simulink model "BBB_USRLED_v2"  (R2013a)
settings: Solver=FixedStepDiscrete  SolverMode=SingleTasking  StartTime=0.0  StopTime=10.0  RelTol=1e-3
libraries: simulink x1
settings Model: ExtModeTrigDuration=100  Creator=rdustinkahawita  LastModifiedBy=rdustinkahawita
settings DataIOCC: InspectSignalLogs=on
settings OptimizationCC: OptimizeModelRefInitCode=on  LifeSpan=1
settings DebuggingCC: SolverPrmCheckMsg=none  StrictBusMsg=Warning
settings HardwareCC: ProdLargestAtomicInteger=Long  ProdLargestAtomicFloat=Double  ProdEndianess=LittleEndian  ProdHWDeviceType=ARM Compatible->ARM Cortex
settings RTWCC: SystemTargetFile=realtime.tlc  GenerateMakefile=off  TemplateMakefile=realtime.tmf  Description=Run on Target Hardware  RTWVerbose=off  ProcessScript=realtime_make_rtw_hook
settings STFCustomTargetCC: TargetLibSuffix=.a  GenerateSampleERTMain=on  ERTCustomFileBanners=on  SupportNonInlinedSFcns=off  SupportVariableSizeSignals=on  MATLABClassNameForMDSCustomization=Simulink.SoftwareTarget.ERTCustomization  SystemTargetFile=realtime.tlc
settings ERTTargetCC: ParMdlRefBuildCompliant=off  CompOptLevelCompliant=off  ConcurrentExecutionCompliant=off  CombineOutputUpdateFcns=off  ERTFirstTimeCompliant=off  SupportContinuousTime=on  SupportVariableSizeSignals=on  ModelStepFunctionPrototypeControlCompliant=off  CPPClassGenCompliant=off  ExtModeMexArgs='192.168.2.14'  ERTSrcFileBannerTemplate=realtime_code_template.cgt  ERTHdrFileBannerTemplate=realtime_code_template.cgt  ERTDataSrcFileTemplate=realtime_code_template.cgt  ERTDataHdrFileTemplate=realtime_code_template.cgt  ERTCustomFileTemplate=realtime_file_process.tlc

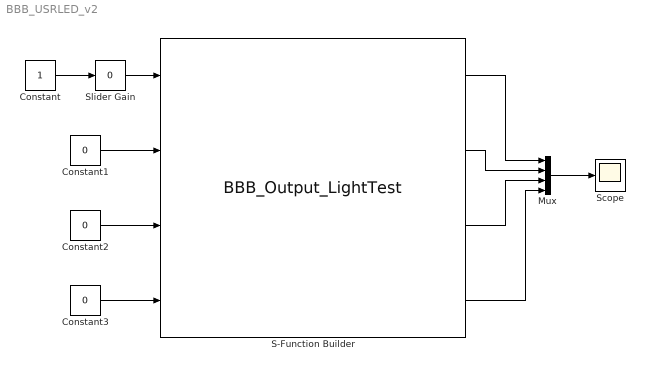
== system BBB_USRLED_v2 ==
  Constant : Constant  OutMin=0  OutMax=1  OutDataTypeStr=boolean  LockScale=on
  Constant1 : Constant  Value=0  OutMin=0  OutMax=1  OutDataTypeStr=boolean  LockScale=on
  Constant2 : Constant  Value=0  OutMin=0  OutMax=1  OutDataTypeStr=boolean  LockScale=on
  Constant3 : Constant  Value=0  OutMin=0  OutMax=1  OutDataTypeStr=boolean  LockScale=on
  Mux : Mux
  S-Function Builder : S-Function  InitFcn=try, set_param(gcb,'FunctionName','BBB_Output_LightTest'), end  FunctionName=BBB_Output_LightTest  Parameters=boolean(0),boolean(0)  SFunctionModules=BBB_Output_LightTest_wrapper  EnableBusSupport=off  mask(S-Function Builder){}
      mask help: Simulink:masks:SFunctionBuilder_MD
      mask init:
      | val = [[.9  0.75 0.75 1 1 .9 .9 1]',[1 1 0.75 0.75 .9 .9 1 .9]'];try , sys = get_param(gcb,'SfunBuilderFcnName');if isempty(sys), sys = get_param(gcb,'FunctionName'); end,catch, sys = get_param(gcb,'FunctionName'); end
      settings: CopyFcn=set_param(gcbh,'LinkStatus','none')  PreSaveFcn=try, set_param(gcb,'FunctionName','BBB_Output_LightTest'), end  OpenFcn=sfunctionwizard(gcbh)
      mask Display: plot(val(:,1),val(:,2)),disp(sys), port_label('input',1,'In_1_LED1'), port_label('input',2,'In_2_LED2'), port_label('input',3,'In_3_LED3'), port_label('input',4,'In_4_LED4'), port_label('output',1,'Out_LED1'), port_label('output',2,'Out_LED2'), port_label('output',3,'Out_LED3'), port_label('output',4,'Out_LED4')
  Scope : Scope
      settings: TimeRange=10
  Slider Gain : simulink/Math Operations/Slider Gain  low=0  gain=0  high=1
  wires:
  Constant/1 -> Slider Gain/1
  Constant1/1 -> S-Function Builder/2
  Constant3/1 -> S-Function Builder/4
  Constant2/1 -> S-Function Builder/3
  S-Function Builder/1 -> Mux/1
  S-Function Builder/2 -> Mux/2
  S-Function Builder/3 -> Mux/3
  S-Function Builder/4 -> Mux/4
  Mux/1 -> Scope/1
  Slider Gain/1 -> S-Function Builder/1
